simulink model "DR_Telemedicine_Workflow"  (R2026a)
settings: Solver=VariableStepAuto

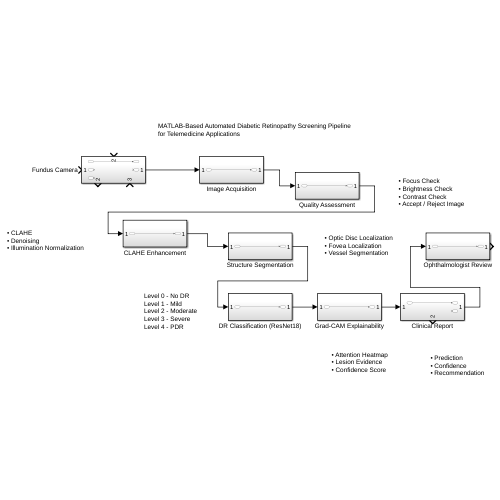
[thumbnail: Simulink's stored preview of the top-level diagram]
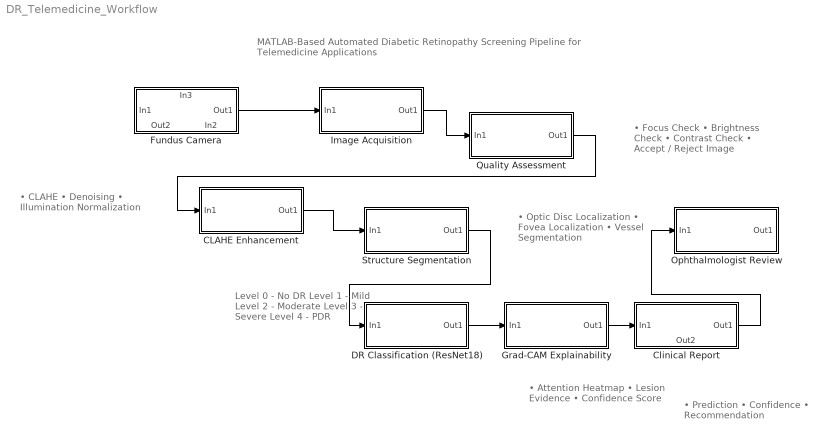
== system DR_Telemedicine_Workflow ==
  note: MATLAB-Based Automated Diabetic Retinopathy Screening Pipeline
      | for Telemedicine Applications
  note: • Prediction
      | • Confidence
      | • Recommendation
  note: • Attention Heatmap
      | • Lesion Evidence
      | • Confidence Score
  note: Level 0 - No DR
      | Level 1 - Mild
      | Level 2 - Moderate
      | Level 3 - Severe
      | Level 4 - PDR
  note: • Optic Disc Localization
      | • Fovea Localization
      | • Vessel Segmentation
  note: • CLAHE
      | • Denoising
      | • Illumination Normalization
  note: • Focus Check
      | • Brightness Check
      | • Contrast Check
      | • Accept / Reject Image
  CLAHE Enhancement : Subsystem
  Clinical Report : Subsystem
      settings: PortSchema="{\"entries\":[{\"content\":{\"sides\":[{\"content\":{\"connectorIds\":[\"In1\"]},\"type\":\"ConnectorPlacement.EquallySpacedRectSide\",\"uuid\":\"7e546d2b-5ec3-44bd-ad4f-190216edd2c7\"},{\"content\":{\"connectorIds\":[\"Out1\"],\"side\":\"RIGHT\"},\"type\":\"ConnectorPlacement.EquallySpacedRectSide\",\"uuid\":\"354e2011-b218-4de8-8d2f-ae67c3941d26\"},{\"content\":{\"side\":\"TOP\"},\"type\":\"ConnectorPlacement.EquallySpacedRectSide\",\"uuid\":\"f91862c8-b4ca-4ed4-8ede-a6bd9fa98302\"},{\"content\":{\"connectorIds\":[\"Out2\"],\"side\":\"BOTTOM\"},\"type\":\"ConnectorPlacement.EquallySpacedRectSide\",\"uuid\":\"0f47aaa5-cc95-4a29-a5e7-4f94ca3f1f63\"}]},\"type\":\"ConnectorPlacement.EquallySpacedConnector\",\"uuid\":\"79c21ace-e02e-4a11-b99d-5e7ab2bfb95b\"}],\"packageUris\":[\"http://schema.mathworks.com/mf0/Connector/R2020b\"],\"version\":\"1.0\"}"
  DR Classification (ResNet18) : Subsystem
  Fundus Camera : Subsystem
      settings: PortSchema="{\"entries\":[{\"content\":{\"sides\":[{\"content\":{\"connectorIds\":[\"In1\"]},\"type\":\"ConnectorPlacement.EquallySpacedRectSide\",\"uuid\":\"7e546d2b-5ec3-44bd-ad4f-190216edd2c7\"},{\"content\":{\"connectorIds\":[\"Out1\"],\"side\":\"RIGHT\"},\"type\":\"ConnectorPlacement.EquallySpacedRectSide\",\"uuid\":\"354e2011-b218-4de8-8d2f-ae67c3941d26\"},{\"content\":{\"connectorIds\":[\"In2\"],\"side\":\"TOP\"},\"type\":\"ConnectorPlacement.EquallySpacedRectSide\",\"uuid\":\"f91862c8-b4ca-4ed4-8ede-a6bd9fa98302\"},{\"content\":{\"connectorIds\":[\"Out2\",\"In3\"],\"side\":\"BOTTOM\"},\"type\":\"ConnectorPlacement.EquallySpacedRectSide\",\"uuid\":\"b84d4432-7ef8-4f61-8b98-13de74de5f93\"}]},\"type\":\"ConnectorPlacement.EquallySpacedConnector\",\"uuid\":\"79c21ace-e02e-4a11-b99d-5e7ab2bfb95b\"}],\"packageUris\":[\"http://schema.mathworks.com/mf0/Connector/R2020b\"],\"version\":\"1.0\"}"
  Grad-CAM Explainability : Subsystem
  Image Acquisition : Subsystem
  Ophthalmologist Review : Subsystem
  Quality Assessment : Subsystem
  Structure Segmentation : Subsystem
  wires:
  Fundus Camera/1(Out1) -> Image Acquisition/1(In1)
  Image Acquisition/1(Out1) -> Quality Assessment/1(In1)
  Quality Assessment/1(Out1) -> CLAHE Enhancement/1(In1)
  CLAHE Enhancement/1(Out1) -> Structure Segmentation/1(In1)
  Structure Segmentation/1(Out1) -> DR Classification (ResNet18)/1(In1)
  DR Classification (ResNet18)/1(Out1) -> Grad-CAM Explainability/1(In1)
  Grad-CAM Explainability/1(Out1) -> Clinical Report/1(In1)
  Clinical Report/1(Out1) -> Ophthalmologist Review/1(In1)

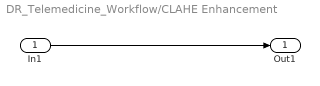
== system DR_Telemedicine_Workflow/CLAHE Enhancement ==
  In1 : Inport
  Out1 : Outport
  wires:
  In1/1 -> Out1/1

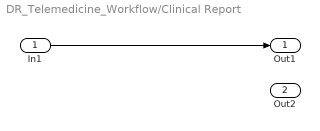
== system DR_Telemedicine_Workflow/Clinical Report ==
  In1 : Inport
  Out1 : Outport
  Out2 : Outport  Port=2
  wires:
  In1/1 -> Out1/1

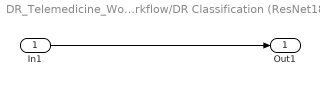
== system DR_Telemedicine_Workflow/DR Classification (ResNet18) ==
  In1 : Inport
  Out1 : Outport
  wires:
  In1/1 -> Out1/1

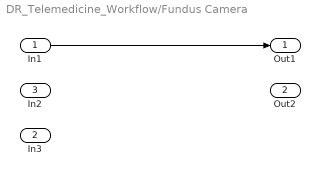
== system DR_Telemedicine_Workflow/Fundus Camera ==
  In1 : Inport
  In3 : Inport  Port=2
  In2 : Inport  Port=3
  Out1 : Outport
  Out2 : Outport  Port=2
  wires:
  In1/1 -> Out1/1

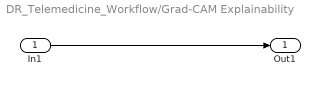
== system DR_Telemedicine_Workflow/Grad-CAM Explainability ==
  In1 : Inport
  Out1 : Outport
  wires:
  In1/1 -> Out1/1

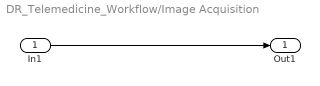
== system DR_Telemedicine_Workflow/Image Acquisition ==
  In1 : Inport
  Out1 : Outport
  wires:
  In1/1 -> Out1/1

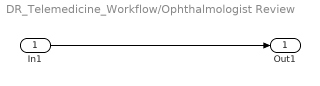
== system DR_Telemedicine_Workflow/Ophthalmologist Review ==
  In1 : Inport
  Out1 : Outport
  wires:
  In1/1 -> Out1/1

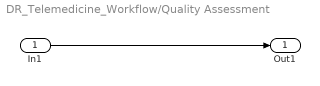
== system DR_Telemedicine_Workflow/Quality Assessment ==
  In1 : Inport
  Out1 : Outport
  wires:
  In1/1 -> Out1/1

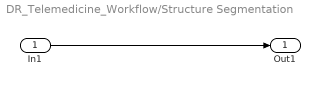
== system DR_Telemedicine_Workflow/Structure Segmentation ==
  In1 : Inport
  Out1 : Outport
  wires:
  In1/1 -> Out1/1
